simulink model "resonatorDiscrete"  (R2025a)
settings: Solver=VariableStepAuto  StartTime=0.0  StopTime=10.0  RelTol=1e-3
values from neighbouring files (symbols this model uses):
  C = 0.001 0.0 0.0 0.001    [resonatorDD.sldd]
  Fd = 1.0    [resonatorDD.sldd]
  K = 1000.0 42.0 23.0 2000.0    [resonatorDD.sldd]
  M = 2.0 0.0 0.0 3.0    [resonatorDD.sldd]
  mc = 1.0    [resonatorDD.sldd]
  om = 0.1    [resonatorDD.sldd]
undefined symbols (not defined in the file or in its folder): DiscIntNeverNeededParam
settings Model: DataDictionary=resonatorDD.sldd  Creator=guirl  LastModifiedBy=guirl

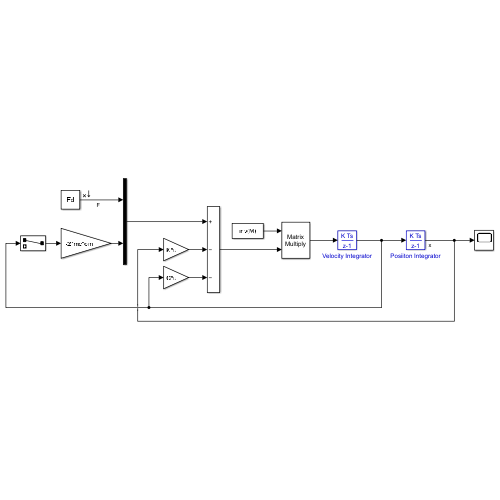
[thumbnail: Simulink's stored preview of the top-level diagram]
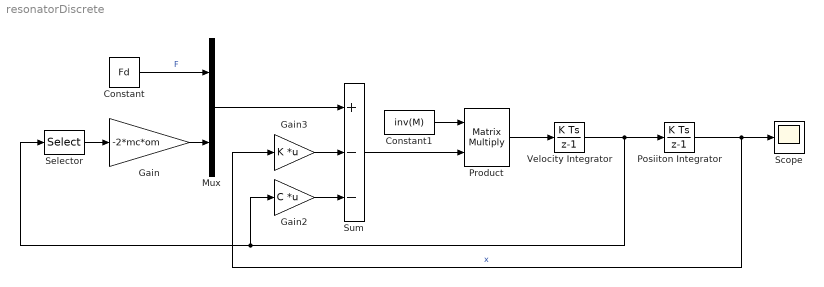
== system resonatorDiscrete ==
  Constant : Constant  Value=Fd
  Constant1 : Constant  Value=inv(M)
  Gain : Gain  Gain=-2*mc*om
  Gain2 : Gain  Gain=C  Multiplication=Matrix(K*u)
  Gain3 : Gain  Gain=K  Multiplication=Matrix(K*u)
  Mux : Mux  Inputs=2
  Posiiton Integrator : DiscreteIntegrator  SampleTime=0.01  ICPrevOutput=DiscIntNeverNeededParam  ICPrevScaledInput=DiscIntNeverNeededParam  mask(DiscretizedDiscreteIntegrator){}
      mask init:
      | %zoh
  Product : Product  Multiplication=Matrix(*)
  Scope : Scope
      settings: ActiveDisplayYMinimum=-0.00044048  ActiveDisplayYMaximum=0.002292  DataLoggingSaveFormat=Array
  Selector : Selector  InputPortWidth=2  IndexOptions=Index vector (dialog)  Indices=1  OutputSizes=1
  Sum : Sum  Inputs=+--
  Velocity Integrator : DiscreteIntegrator  SampleTime=0.01  ICPrevOutput=DiscIntNeverNeededParam  ICPrevScaledInput=DiscIntNeverNeededParam  mask(DiscretizedDiscreteIntegrator){}
      mask init:
      | %zoh
  wires:
  Constant1/1 -> Product/1
  Selector/1 -> Gain/1
  Sum/1 -> Product/2
  Gain2/1 -> Sum/3
  Gain3/1 -> Sum/2
  Mux/1 -> Sum/1
  Velocity Integrator/1 -> Selector/1, Gain2/1, Posiiton Integrator/1
  Posiiton Integrator/1 -> Scope/1, Gain3/1  "x"
  Product/1 -> Velocity Integrator/1
  Gain/1 -> Mux/2
  Constant/1 -> Mux/1  "F"
